simulink library "INT_EnvT_VD"  (R2016b)
settings: Solver=VariableStepAuto  StartTime=0.0  StopTime=10.0  RelTol=1e-3
settings Model: Creator=Administrator  LastModifiedBy=Administrator

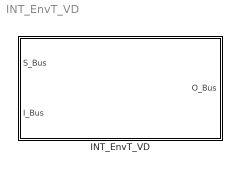
== system INT_EnvT_VD ==
  INT_EnvT_VD : Subsystem

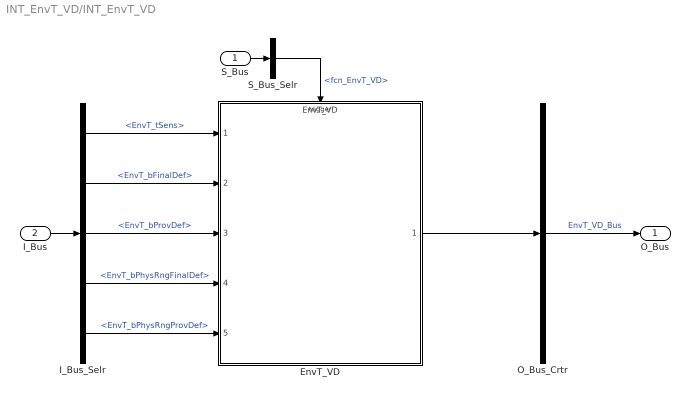
== system INT_EnvT_VD/INT_EnvT_VD ==
  S_Bus : Inport
  I_Bus : Inport  Port=2
  EnvT_VD : ModelReference  ModelNameDialog=EnvT_VD  SimulationMode=Normal  ModelReferenceVersion=1.8  TriggerPortName=function  TriggerPortTriggerType=function-call  TriggerPortStatesWhenEnabling=held
  I_Bus_Selr : BusSelector  OutputSignals=EnvT_tSens,EnvT_bFinalDef,EnvT_bProvDef,EnvT_bPhysRngFinalDef,EnvT_bPhysRngProvDef
  O_Bus_Crtr : BusCreator  Inputs=1
  S_Bus_Selr : BusSelector  OutputSignals=fcn_EnvT_VD
  O_Bus : Outport
  wires:
  S_Bus_Selr/1 -> EnvT_VD/Trigger  "<fcn_EnvT_VD>"
  S_Bus/1 -> S_Bus_Selr/1
  I_Bus/1 -> I_Bus_Selr/1
  I_Bus_Selr/1 -> EnvT_VD/1  "<EnvT_tSens>"
  I_Bus_Selr/2 -> EnvT_VD/2  "<EnvT_bFinalDef>"
  I_Bus_Selr/3 -> EnvT_VD/3  "<EnvT_bProvDef>"
  I_Bus_Selr/4 -> EnvT_VD/4  "<EnvT_bPhysRngFinalDef>"
  I_Bus_Selr/5 -> EnvT_VD/5  "<EnvT_bPhysRngProvDef>"
  O_Bus_Crtr/1 -> O_Bus/1  "EnvT_VD_Bus"
  EnvT_VD/1 -> O_Bus_Crtr/1
